simulink model "cc_simulink"  (R2023a)
settings: Solver=VariableStepAuto  StartTime=0.0  StopTime=5100  RelTol=1e-3
undefined symbols (not defined in the file): g_i, g_p
libraries: simulink x6, hdlsllib x1
settings Model: Creator=usradmin  LastModifiedBy=harry

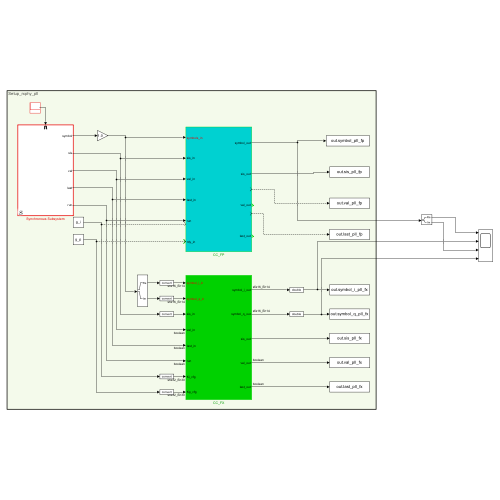
[thumbnail: Simulink's stored preview of the top-level diagram]
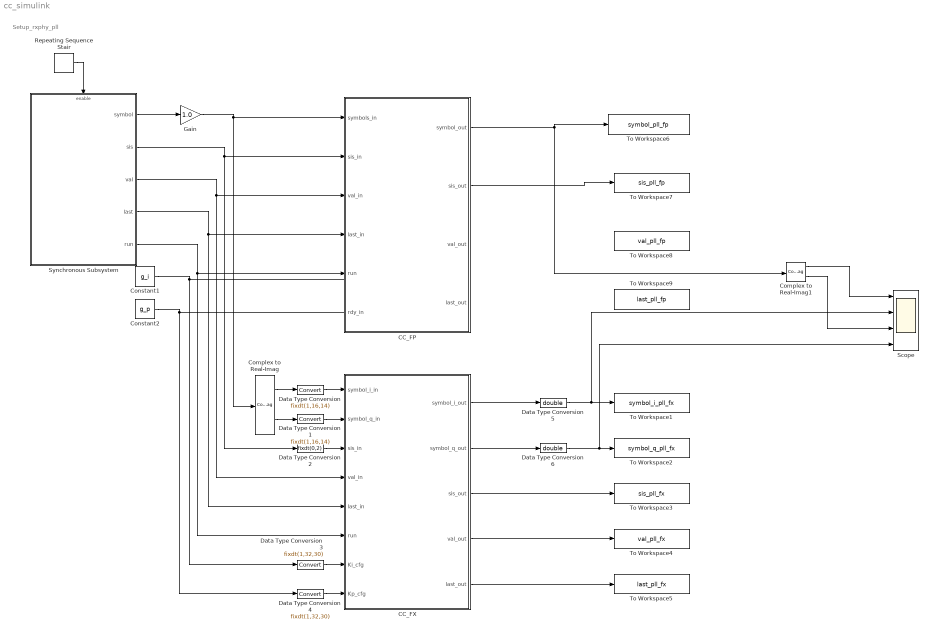
== system cc_simulink ==
  note: Setup_rxphy_pll
  CC_FP : Subsystem
  CC_FX : Subsystem
  Complex to Real-Imag : ComplexToRealImag
  Complex to Real-Imag1 : ComplexToRealImag
  Constant1 : Constant  Value=g_i  SampleTime=-1
  Constant2 : Constant  Value=g_p  SampleTime=-1
  Data Type Conversion : DataTypeConversion  OutDataTypeStr=fixdt(1,16,14)  SaturateOnIntegerOverflow=off  RndMeth=Floor
  Data Type Conversion1 : DataTypeConversion  OutDataTypeStr=fixdt(1,16,14)  SaturateOnIntegerOverflow=off  RndMeth=Floor
  Data Type Conversion2 : DataTypeConversion  OutMin=[0]  OutMax=[3]  OutDataTypeStr=fixdt(0,2)  SaturateOnIntegerOverflow=off  RndMeth=Floor
  Data Type Conversion3 : DataTypeConversion  OutDataTypeStr=fixdt(1,32,30)  SaturateOnIntegerOverflow=off  RndMeth=Floor
  Data Type Conversion4 : DataTypeConversion  OutDataTypeStr=fixdt(1,32,30)  SaturateOnIntegerOverflow=off  RndMeth=Floor
  Data Type Conversion5 : DataTypeConversion  OutDataTypeStr=double  SaturateOnIntegerOverflow=off  RndMeth=Floor
  Data Type Conversion6 : DataTypeConversion  OutDataTypeStr=double  SaturateOnIntegerOverflow=off  RndMeth=Floor
  Gain : Gain  Gain=1.0
  Repeating Sequence Stair : simulink/Sources/Repeating Sequence Stair  OutValues=1  tsamp=1  OutMin=[]  OutMax=[]  OutDataTypeStr=double  OutputDataTypeScalingMode=double  OutDataType=fixdt(0,8)  ConRadixGroup=Best Precision: Vector-wise  OutScaling=2^-12
  Scope : Scope  NumInputPorts=4
  Synchronous Subsystem : Subsystem
  To Workspace1 : ToWorkspace  VariableName=symbol_i_pll_fx  SampleTime=-1
      settings: Save2DSignal=2-D array (concatenate along first dimension)
  To Workspace2 : ToWorkspace  VariableName=symbol_q_pll_fx  SampleTime=-1
      settings: Save2DSignal=2-D array (concatenate along first dimension)
  To Workspace3 : ToWorkspace  VariableName=sis_pll_fx  SampleTime=-1
      settings: Save2DSignal=2-D array (concatenate along first dimension)
  To Workspace4 : ToWorkspace  VariableName=val_pll_fx  SampleTime=-1
      settings: Save2DSignal=2-D array (concatenate along first dimension)
  To Workspace5 : ToWorkspace  VariableName=last_pll_fx  SampleTime=-1
      settings: Save2DSignal=2-D array (concatenate along first dimension)
  To Workspace6 : ToWorkspace  VariableName=symbol_pll_fp  SampleTime=-1
      settings: Save2DSignal=2-D array (concatenate along first dimension)
  To Workspace7 : ToWorkspace  VariableName=sis_pll_fp  SampleTime=-1
      settings: Save2DSignal=2-D array (concatenate along first dimension)
  To Workspace8 : ToWorkspace  VariableName=val_pll_fp  SampleTime=-1
      settings: Save2DSignal=2-D array (concatenate along first dimension)
  To Workspace9 : ToWorkspace  VariableName=last_pll_fp  SampleTime=-1
      settings: Save2DSignal=2-D array (concatenate along first dimension)
  wires:
  Repeating Sequence Stair/1 -> Synchronous Subsystem/Enable
  Synchronous Subsystem/1(symbol) -> Gain/1
  Synchronous Subsystem/4(last) -> CC_FX/5(last_in), CC_FP/4(last_in)
  ? -> To Workspace8/1
  ? -> To Workspace9/1
  Constant1/1 -> Data Type Conversion3/1
  Constant2/1 -> Data Type Conversion4/1
  Synchronous Subsystem/2(sis) -> Data Type Conversion2/1, CC_FP/2(sis_in)
  Synchronous Subsystem/5(run) -> CC_FX/6(run), CC_FP/5(run)
  Synchronous Subsystem/3(val) -> CC_FX/4(val_in), CC_FP/3(val_in)
  CC_FP/2(sis_out) -> To Workspace7/1
  CC_FP/1(symbol_out) -> Complex to Real-Imag1/1, To Workspace6/1
  Data Type Conversion3/1 -> CC_FX/7(Ki_cfg)
  Data Type Conversion4/1 -> CC_FX/8(Kp_cfg)
  Data Type Conversion/1 -> CC_FX/1(symbol_i_in)
  Data Type Conversion1/1 -> CC_FX/2(symbol_q_in)
  Data Type Conversion2/1 -> CC_FX/3(sis_in)
  Complex to Real-Imag/1 -> Data Type Conversion/1
  Complex to Real-Imag/2 -> Data Type Conversion1/1
  CC_FX/1(symbol_i_out) -> Data Type Conversion5/1
  Data Type Conversion5/1 -> Scope/2, To Workspace1/1
  CC_FX/2(symbol_q_out) -> Data Type Conversion6/1
  Data Type Conversion6/1 -> Scope/4, To Workspace2/1
  CC_FX/3(sis_out) -> To Workspace3/1
  CC_FX/4(val_out) -> To Workspace4/1
  CC_FX/5(last_out) -> To Workspace5/1
  Gain/1 -> Complex to Real-Imag/1, CC_FP/1(symbols_in)
  Complex to Real-Imag1/1 -> Scope/1
  Complex to Real-Imag1/2 -> Scope/3

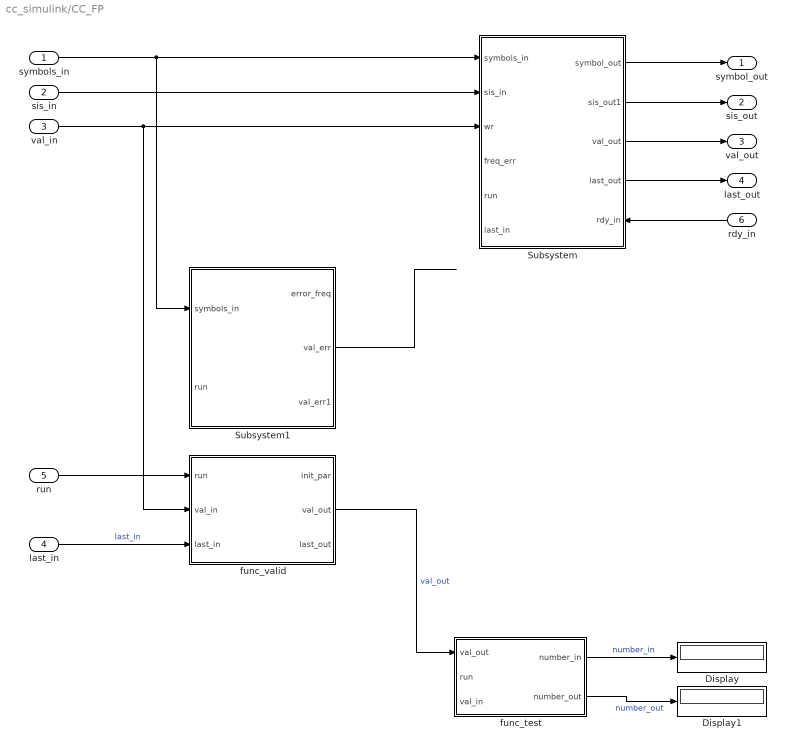
== system cc_simulink/CC_FP ==
  symbols_in : Inport
  sis_in : Inport  Port=2
  val_in : Inport  Port=3
  last_in : Inport  Port=4
  run : Inport  Port=5
  rdy_in : Inport  Port=6
  Display : Display
  Display1 : Display
  Subsystem : Subsystem
      settings: PortSchema="{\"entries\":[{\"content\":{\"sides\":[{\"content\":{\"connectorIds\":[\"In1\",\"In2\",\"In3\",\"In4\",\"In5\",\"In6\"]},\"type\":\"ConnectorPlacement.EquallySpacedRectSide\",\"uuid\":\"c7939d33-c946-4bf1-9bdf-2b3408225bc2\"},{\"content\":{\"connectorIds\":[\"Out1\",\"Out2\",\"Out3\",\"Out4\",\"In7\"],\"side\":\"RIGHT\"},\"type\":\"ConnectorPlacement.EquallySpacedRectSide\",\"uuid\":\"307b9761-00b9-4204-91fa-5162dfa483c4\"},{\"content\":{\"side\":\"TOP\"},\"type\":\"ConnectorPlacement.EquallySpacedRectSide\",\"uuid\":\"84444ae4-1671-4931-bee6-6f05b65457b7\"}]},\"type\":\"ConnectorPlacement.EquallySpacedConnector\",\"uuid\":\"d9ea343b-4c68-49a2-bcf3-6268f7ae1a01\"}],\"packageUris\":[\"http://schema.mathworks.com/mf0/Connector/R2020b\"],\"version\":\"1.0\"}"
  Subsystem1 : Subsystem
  func_test : MATLAB Function  TreatAsAtomicUnit=on
  func_valid : MATLAB Function  TreatAsAtomicUnit=on
  symbol_out : Outport
  sis_out : Outport  Port=2
  val_out : Outport  Port=3
  last_out : Outport  Port=4
  wires:
  val_in/1 -> func_valid/2(val_in), Subsystem/3(wr)
  last_in/1 -> func_valid/3(last_in)  "last_in"
  func_valid/2(val_out) -> func_test/1(val_out)  "val_out"
  run/1 -> func_valid/1(run)
  func_test/1(number_in) -> Display/1  "number_in"
  func_test/2(number_out) -> Display1/1  "number_out"
  symbols_in/1 -> Subsystem1/1(symbols_in), Subsystem/1(symbols_in)
  sis_in/1 -> Subsystem/2(sis_in)
  Subsystem/2(sis_out1) -> sis_out/1
  Subsystem1/2(val_err) -> ?
  Subsystem/1(symbol_out) -> symbol_out/1
  Subsystem/3(val_out) -> val_out/1
  Subsystem/4(last_out) -> last_out/1
  rdy_in/1 -> Subsystem/7(rdy_in)

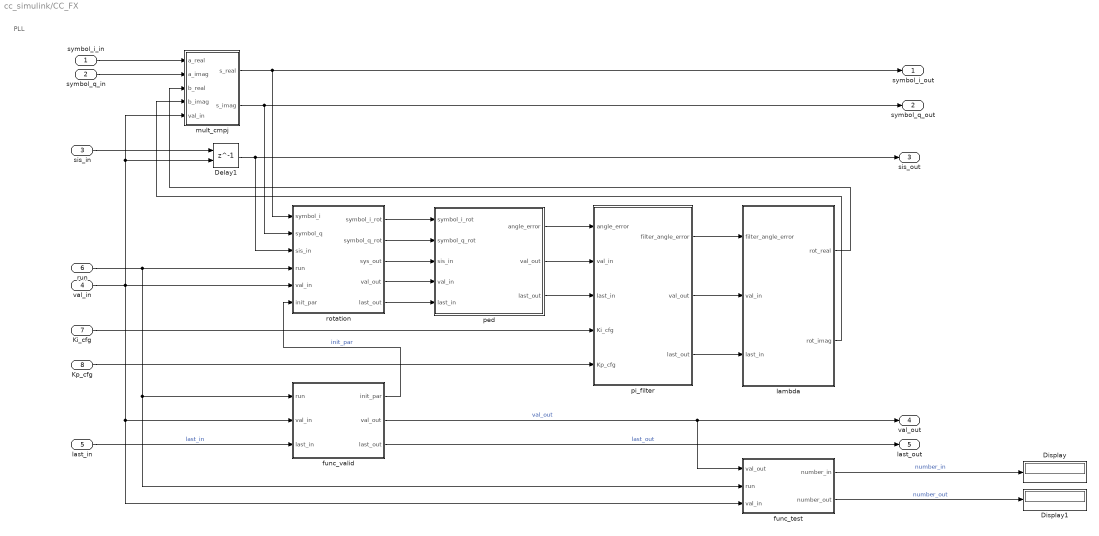
== system cc_simulink/CC_FX ==
  note: PLL
  symbol_i_in : Inport  OutDataTypeStr=fixdt(1,16,14)
  symbol_q_in : Inport  Port=2  OutDataTypeStr=fixdt(1,16,14)
  sis_in : Inport  Port=3  OutMin=[0]  OutMax=[3]  OutDataTypeStr=fixdt(0,2)
  val_in : Inport  Port=4  OutDataTypeStr=boolean
  last_in : Inport  Port=5  OutDataTypeStr=boolean
  run : Inport  Port=6  OutDataTypeStr=boolean
  Ki_cfg : Inport  Port=7  OutDataTypeStr=fixdt(1,32,30)
  Kp_cfg : Inport  Port=8  OutDataTypeStr=fixdt(1,32,30)
  Delay1 : Delay  DelayLength=1  InitialCondition=0  ShowEnablePort=on
      settings: InputPortMap=u0,e6
  Display : Display
  Display1 : Display
  func_test : MATLAB Function  TreatAsAtomicUnit=on
  func_valid : MATLAB Function  TreatAsAtomicUnit=on
  lambda : Subsystem
  mult_cmpj : Subsystem
  ped : Subsystem
  pi_filter : Subsystem
  rotation : Subsystem
  symbol_i_out : Outport  OutDataTypeStr=fixdt(1,16,14)
  symbol_q_out : Outport  Port=2  OutDataTypeStr=fixdt(1,16,14)
  sis_out : Outport  Port=3  OutMin=[0]  OutMax=[3]  OutDataTypeStr=fixdt(0,2)
  val_out : Outport  Port=4  OutDataTypeStr=boolean
  last_out : Outport  Port=5  OutDataTypeStr=boolean
  wires:
  func_test/2(number_out) -> Display1/1  "number_out"
  func_test/1(number_in) -> Display/1  "number_in"
  symbol_i_in/1 -> mult_cmpj/1(a_real)
  func_valid/1(init_par) -> rotation/6(init_par)  "init_par"
  Delay1/1 -> rotation/3(sis_in), sis_out/1
  run/1 -> rotation/4(run), func_valid/1(run), func_test/2(run)
  Kp_cfg/1 -> pi_filter/5(Kp_cfg)
  Ki_cfg/1 -> pi_filter/4(Ki_cfg)
  func_valid/3(last_out) -> last_out/1  "last_out"
  func_valid/2(val_out) -> func_test/1(val_out), val_out/1  "val_out"
  mult_cmpj/1(s_real) -> rotation/1(symbol_i), symbol_i_out/1
  pi_filter/3(last_out) -> lambda/3(last_in)
  pi_filter/2(val_out) -> lambda/2(val_in)
  ped/3(last_out) -> pi_filter/3(last_in)
  ped/2(val_out) -> pi_filter/2(val_in)
  rotation/5(last_out) -> ped/5(last_in)
  rotation/4(val_out) -> ped/4(val_in)
  last_in/1 -> func_valid/3(last_in)  "last_in"
  val_in/1 -> mult_cmpj/5(val_in), Delay1/2, rotation/5(val_in), func_valid/2(val_in), func_test/3(val_in)
  rotation/3(sys_out) -> ped/3(sis_in)
  sis_in/1 -> Delay1/1
  pi_filter/1(filter_angle_error) -> lambda/1(filter_angle_error)
  ped/1(angle_error) -> pi_filter/1(angle_error)
  symbol_q_in/1 -> mult_cmpj/2(a_imag)
  mult_cmpj/2(s_imag) -> symbol_q_out/1, rotation/2(symbol_q)
  rotation/1(symbol_i_rot) -> ped/1(symbol_i_rot)
  rotation/2(symbol_q_rot) -> ped/2(symbol_q_rot)
  lambda/1(rot_real) -> mult_cmpj/3(b_real)
  lambda/2(rot_imag) -> mult_cmpj/4(b_imag)

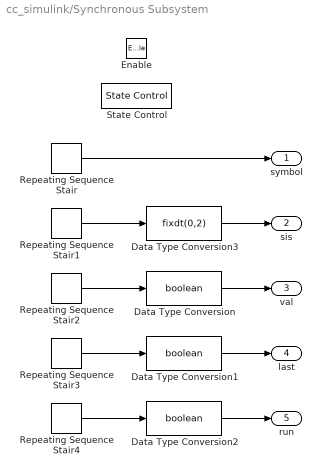
== system cc_simulink/Synchronous Subsystem ==
  Enable : EnablePort  ShowOutputPort=on
  Data Type Conversion : DataTypeConversion  OutDataTypeStr=boolean  SaturateOnIntegerOverflow=off  RndMeth=Floor
  Data Type Conversion1 : DataTypeConversion  OutDataTypeStr=boolean  SaturateOnIntegerOverflow=off  RndMeth=Floor
  Data Type Conversion2 : DataTypeConversion  OutDataTypeStr=boolean  SaturateOnIntegerOverflow=off  RndMeth=Floor
  Data Type Conversion3 : DataTypeConversion  OutMin=[0]  OutMax=[3]  OutDataTypeStr=fixdt(0,2)  SaturateOnIntegerOverflow=off  RndMeth=Floor
  Repeating Sequence Stair : simulink/Sources/Repeating Sequence Stair  OutValues=symbols_cc  tsamp=1  OutMin=[]  OutMax=[]  OutDataTypeStr=double  OutputDataTypeScalingMode=double  OutDataType=fixdt(0,8)  ConRadixGroup=Best Precision: Vector-wise  OutScaling=2^-12
  Repeating Sequence Stair1 : simulink/Sources/Repeating Sequence Stair  OutValues=sis_cc  tsamp=1  OutMin=[]  OutMax=[]  OutDataTypeStr=double  OutputDataTypeScalingMode=double  OutDataType=fixdt(0,8)  ConRadixGroup=Best Precision: Vector-wise  OutScaling=2^-12
  Repeating Sequence Stair2 : simulink/Sources/Repeating Sequence Stair  OutValues=val_cc  tsamp=1  OutMin=[]  OutMax=[]  OutDataTypeStr=double  OutputDataTypeScalingMode=double  OutDataType=fixdt(0,8)  ConRadixGroup=Best Precision: Vector-wise  OutScaling=2^-12
  Repeating Sequence Stair3 : simulink/Sources/Repeating Sequence Stair  OutValues=last_cc  tsamp=1  OutMin=[]  OutMax=[]  OutDataTypeStr=double  OutputDataTypeScalingMode=double  OutDataType=fixdt(0,8)  ConRadixGroup=Best Precision: Vector-wise  OutScaling=2^-12
  Repeating Sequence Stair4 : simulink/Sources/Repeating Sequence Stair  OutValues=run_cc  tsamp=1  OutMin=[]  OutMax=[]  OutDataTypeStr=double  OutputDataTypeScalingMode=double  OutDataType=fixdt(0,8)  ConRadixGroup=Best Precision: Vector-wise  OutScaling=2^-12
  State Control : StateControl  StateControl=Synchronous
  symbol : Outport  VectorParamsAs1DForOutWhenUnconnected=off
  sis : Outport  Port=2  VectorParamsAs1DForOutWhenUnconnected=off
  val : Outport  Port=3  VectorParamsAs1DForOutWhenUnconnected=off
  last : Outport  Port=4  VectorParamsAs1DForOutWhenUnconnected=off
  run : Outport  Port=5  VectorParamsAs1DForOutWhenUnconnected=off
  wires:
  Repeating Sequence Stair/1 -> symbol/1
  Repeating Sequence Stair1/1 -> Data Type Conversion3/1
  Repeating Sequence Stair3/1 -> Data Type Conversion1/1
  Repeating Sequence Stair2/1 -> Data Type Conversion/1
  Repeating Sequence Stair4/1 -> Data Type Conversion2/1
  Data Type Conversion/1 -> val/1
  Data Type Conversion1/1 -> last/1
  Data Type Conversion2/1 -> run/1
  Data Type Conversion3/1 -> sis/1

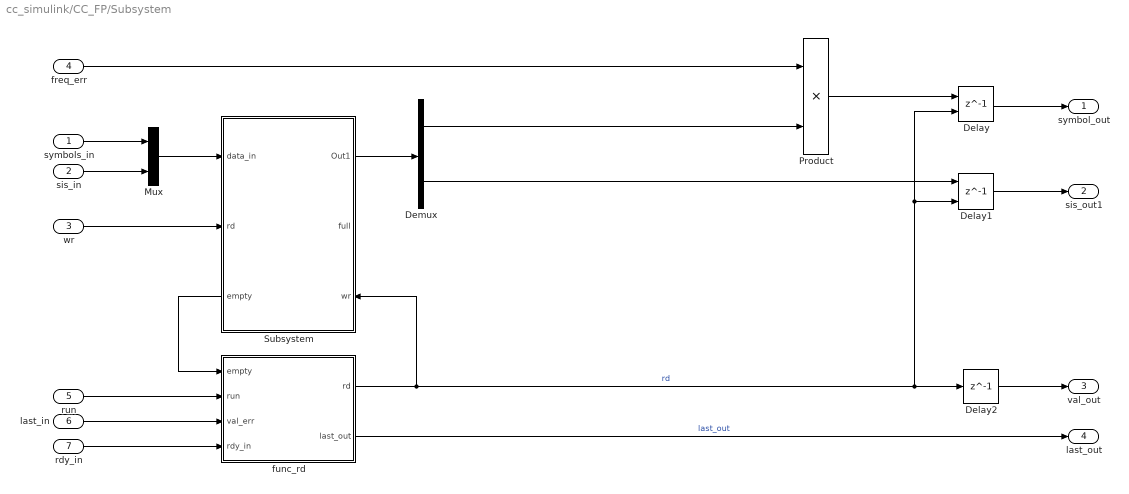
== system cc_simulink/CC_FP/Subsystem ==
  symbols_in : Inport
  sis_in : Inport  Port=2
  wr : Inport  Port=3
  freq_err : Inport  Port=4
  run : Inport  Port=5
  last_in : Inport  Port=6
  rdy_in : Inport  Port=7
  Delay : Delay  DelayLength=1  InitialCondition=0  ShowEnablePort=on
      settings: InputPortMap=u0,e6
  Delay1 : Delay  DelayLength=1  InitialCondition=0  ShowEnablePort=on
      settings: InputPortMap=u0,e6
  Delay2 : Delay  DelayLength=1  InitialCondition=0
  Demux : Demux  Outputs=2
  Mux : Mux  Inputs=2
  Product : Product
  Subsystem : Subsystem
      settings: PortSchema="{\"entries\":[{\"content\":{\"sides\":[{\"content\":{\"connectorIds\":[\"In1\",\"In2\",\"Out3\"]},\"type\":\"ConnectorPlacement.EquallySpacedRectSide\",\"uuid\":\"bfd53dd1-7a31-4f51-b3c2-6d63477d1785\"},{\"content\":{\"connectorIds\":[\"Out1\",\"Out2\",\"In3\"],\"side\":\"RIGHT\"},\"type\":\"ConnectorPlacement.EquallySpacedRectSide\",\"uuid\":\"4f2d7eeb-26ef-45c7-bd9a-3a631e6797b8\"},{\"content\":{\"side\":\"TOP\"},\"type\":\"ConnectorPlacement.EquallySpacedRectSide\",\"uuid\":\"17e64bb6-dd6a-4970-b765-577857b607e2\"}]},\"type\":\"ConnectorPlacement.EquallySpacedConnector\",\"uuid\":\"4ca766b8-8fb8-4689-a29d-3d913e337836\"}],\"packageUris\":[\"http://schema.mathworks.com/mf0/Connector/R2020b\"],\"version\":\"1.0\"}"
  func_rd : MATLAB Function  TreatAsAtomicUnit=on
  symbol_out : Outport
  sis_out1 : Outport  Port=2
  val_out : Outport  Port=3
  last_out : Outport  Port=4
  wires:
  symbols_in/1 -> Mux/1
  sis_in/1 -> Mux/2
  Delay2/1 -> val_out/1
  Delay1/1 -> sis_out1/1
  Product/1 -> Delay/1
  Demux/2 -> Delay1/1
  Delay/1 -> symbol_out/1
  func_rd/1(rd) -> Subsystem/3(wr), Delay/2, Delay1/2, Delay2/1  "rd"
  Demux/1 -> Product/2
  freq_err/1 -> Product/1
  run/1 -> func_rd/2(run)
  func_rd/2(last_out) -> last_out/1  "last_out"
  Mux/1 -> Subsystem/1(data_in)
  wr/1 -> Subsystem/2(rd)
  Subsystem/1(Out1) -> Demux/1
  Subsystem/3(empty) -> func_rd/1(empty)
  last_in/1 -> func_rd/3(val_err)
  rdy_in/1 -> func_rd/4(rdy_in)

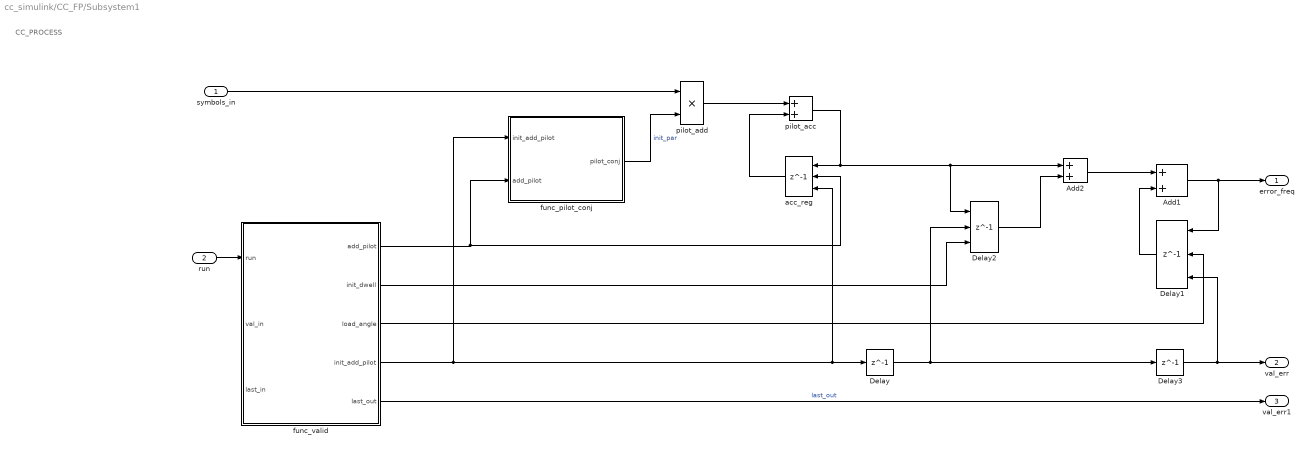
== system cc_simulink/CC_FP/Subsystem1 ==
  note: CC_PROCESS
  symbols_in : Inport
  run : Inport  Port=2
  Add1 : Sum
  Add2 : Sum
  Delay : Delay  DelayLength=1  InitialCondition=0
  Delay1 : Delay  DelayLength=1  InitialCondition=0  ExternalReset=Level  ShowEnablePort=on
      settings: InputPortMap=u0,e6,r5
  Delay2 : Delay  DelayLength=1  InitialCondition=0  ExternalReset=Level  ShowEnablePort=on
      settings: InputPortMap=u0,e6,r5
  Delay3 : Delay  DelayLength=1  InitialCondition=0
  acc_reg : Delay  DelayLength=1  InitialCondition=0  ExternalReset=Level  ShowEnablePort=on
      settings: InputPortMap=u0,e6,r5
  func_pilot_conj : MATLAB Function  TreatAsAtomicUnit=on
  func_valid : MATLAB Function  TreatAsAtomicUnit=on
  pilot_acc : Sum
  pilot_add : Product
  error_freq : Outport
  val_err : Outport  Port=2
  val_err1 : Outport  Port=3
  wires:
  pilot_acc/1 -> Add2/1, Delay2/1, acc_reg/1
  Delay2/1 -> Add2/2
  Delay1/1 -> Add1/2
  Add1/1 -> Delay1/1, error_freq/1
  Add2/1 -> Add1/1
  acc_reg/1 -> pilot_acc/2
  func_valid/1(add_pilot) -> func_pilot_conj/2(add_pilot), acc_reg/2
  func_valid/3(load_angle) -> Delay1/2
  func_valid/4(init_add_pilot) -> acc_reg/3, Delay/1, func_pilot_conj/1(init_add_pilot)
  symbols_in/1 -> pilot_add/1
  pilot_add/1 -> pilot_acc/1
  func_pilot_conj/1(pilot_conj) -> pilot_add/2  "init_par"
  Delay/1 -> Delay3/1, Delay2/2
  func_valid/2(init_dwell) -> Delay2/3
  Delay3/1 -> val_err/1, Delay1/3
  run/1 -> func_valid/1(run)
  func_valid/5(last_out) -> val_err1/1  "last_out"

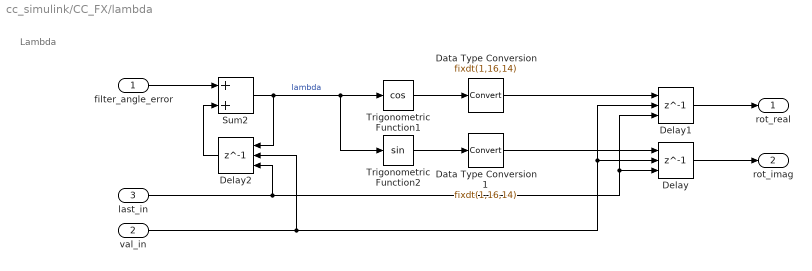
== system cc_simulink/CC_FX/lambda ==
  note: Lambda
  filter_angle_error : Inport
  val_in : Inport  Port=2
  last_in : Inport  Port=3
  Data Type Conversion : DataTypeConversion  OutDataTypeStr=fixdt(1,16,14)  SaturateOnIntegerOverflow=off  RndMeth=Floor
  Data Type Conversion1 : DataTypeConversion  OutDataTypeStr=fixdt(1,16,14)  SaturateOnIntegerOverflow=off  RndMeth=Floor
  Delay : Delay  DelayLength=1  InitialCondition=0  ExternalReset=Level  ShowEnablePort=on
      settings: InputPortMap=u0,e6,r5
  Delay1 : Delay  DelayLength=1  InitialCondition=0  ExternalReset=Level  ShowEnablePort=on
      settings: InputPortMap=u0,e6,r5
  Delay2 : Delay  DelayLength=1  ExternalReset=Level  ShowEnablePort=on
      settings: InputPortMap=u0,e6,r5
  Sum2 : Sum  AccumDataTypeStr=fixdt(1,24,20)
  Trigonometric Function1 : Trigonometry  Operator=cos  ApproximationMethod=Lookup  NumberOfDataPoints=2048  TableDataTypeStr=fixdt(1,12,10)
  Trigonometric Function2 : Trigonometry  ApproximationMethod=Lookup  NumberOfDataPoints=4096  TableDataTypeStr=fixdt(1,12,10)
  rot_real : Outport
  rot_imag : Outport  Port=2
  wires:
  Trigonometric Function1/1 -> Data Type Conversion/1
  Trigonometric Function2/1 -> Data Type Conversion1/1
  Delay/1 -> rot_imag/1
  val_in/1 -> Delay2/2, Delay1/2, Delay/2
  last_in/1 -> Delay2/3, Delay1/3, Delay/3
  filter_angle_error/1 -> Sum2/1
  Delay2/1 -> Sum2/2
  Sum2/1 -> Delay2/1, Trigonometric Function2/1, Trigonometric Function1/1  "lambda"
  Data Type Conversion/1 -> Delay1/1
  Data Type Conversion1/1 -> Delay/1
  Delay1/1 -> rot_real/1

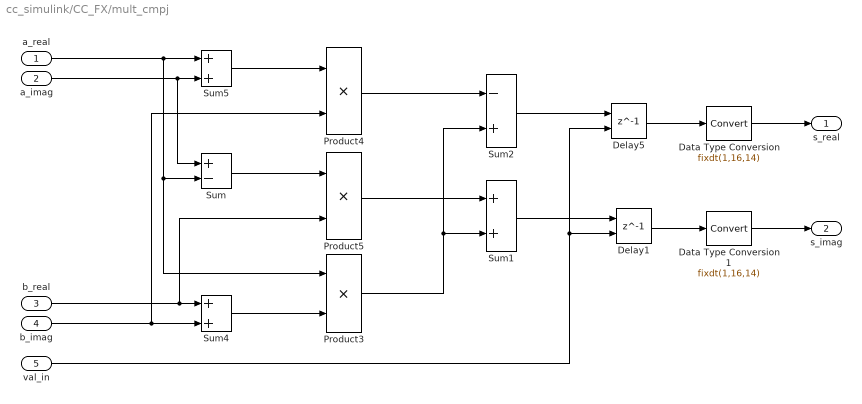
== system cc_simulink/CC_FX/mult_cmpj ==
  a_real : Inport
  a_imag : Inport  Port=2
  b_real : Inport  Port=3
  b_imag : Inport  Port=4
  val_in : Inport  Port=5
  Data Type Conversion : DataTypeConversion  OutDataTypeStr=fixdt(1,16,14)  SaturateOnIntegerOverflow=off  RndMeth=Floor
  Data Type Conversion1 : DataTypeConversion  OutDataTypeStr=fixdt(1,16,14)  SaturateOnIntegerOverflow=off  RndMeth=Floor
  Delay1 : Delay  DelayLength=1  InitialCondition=0  ShowEnablePort=on
      settings: InputPortMap=u0,e6
  Delay5 : Delay  DelayLength=1  InitialCondition=0  ShowEnablePort=on
      settings: InputPortMap=u0,e6
  Product3 : Product
  Product4 : Product
  Product5 : Product
  Sum : Sum  Inputs=+-
  Sum1 : Sum
  Sum2 : Sum  Inputs=-+
  Sum4 : Sum
  Sum5 : Sum
  s_real : Outport
  s_imag : Outport  Port=2
  wires:
  Product3/1 -> Sum1/2, Sum2/2
  Sum1/1 -> Delay1/1
  b_real/1 -> Sum4/1, Product5/2
  Sum2/1 -> Delay5/1
  a_real/1 -> Sum5/1, Product3/1, Sum/2
  b_imag/1 -> Sum4/2, Product4/2
  a_imag/1 -> Sum/1, Sum5/2
  Sum4/1 -> Product3/2
  Sum5/1 -> Product4/1
  Sum/1 -> Product5/1
  Product4/1 -> Sum2/1
  Product5/1 -> Sum1/1
  Delay5/1 -> Data Type Conversion/1
  Delay1/1 -> Data Type Conversion1/1
  val_in/1 -> Delay5/2, Delay1/2
  Data Type Conversion/1 -> s_real/1
  Data Type Conversion1/1 -> s_imag/1

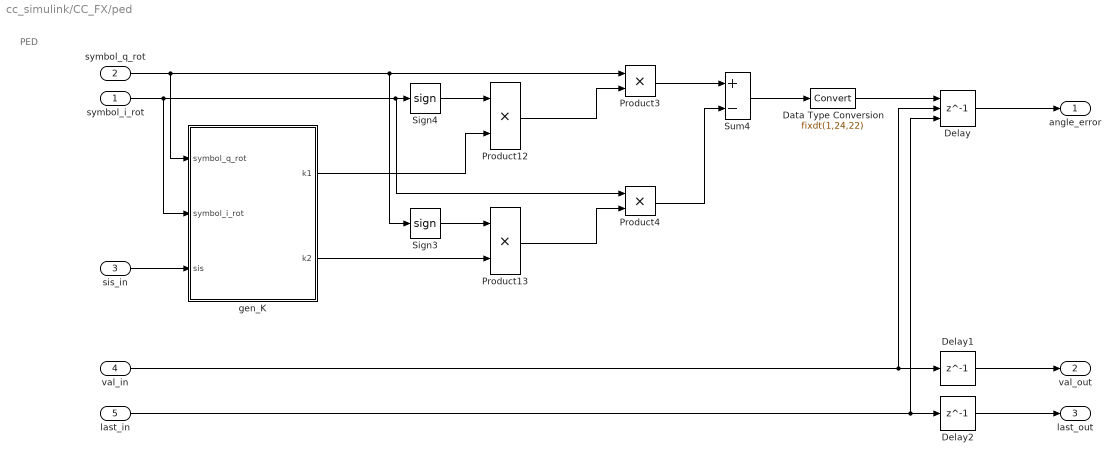
== system cc_simulink/CC_FX/ped ==
  note: PED
  symbol_i_rot : Inport
  symbol_q_rot : Inport  Port=2
  sis_in : Inport  Port=3
  val_in : Inport  Port=4
  last_in : Inport  Port=5
  Data Type Conversion : DataTypeConversion  OutDataTypeStr=fixdt(1,24,22)  SaturateOnIntegerOverflow=off  RndMeth=Floor
  Delay : Delay  DelayLength=1  InitialCondition=0  ExternalReset=Level  ShowEnablePort=on
      settings: InputPortMap=u0,e6,r5
  Delay1 : Delay  DelayLength=1  InitialCondition=0
  Delay2 : Delay  DelayLength=1  InitialCondition=0
  Product{3..4,12..13} (4 alike) : Product
  Sign3 : Signum
  Sign4 : Signum
  Sum4 : Sum  Inputs=+-
  gen_K : MATLAB Function  TreatAsAtomicUnit=on
  angle_error : Outport
  val_out : Outport  Port=2
  last_out : Outport  Port=3
  wires:
  gen_K/2(k2) -> Product13/2
  last_in/1 -> Delay/3, Delay2/1
  val_in/1 -> Delay1/1, Delay/2
  sis_in/1 -> gen_K/3(sis)
  Product13/1 -> Product4/2
  symbol_q_rot/1 -> gen_K/1(symbol_q_rot), Product3/1, Sign3/1
  Sign4/1 -> Product12/1
  Sign3/1 -> Product13/1
  Product4/1 -> Sum4/2
  Sum4/1 -> Data Type Conversion/1
  gen_K/1(k1) -> Product12/2
  Product12/1 -> Product3/2
  Product3/1 -> Sum4/1
  symbol_i_rot/1 -> gen_K/2(symbol_i_rot), Product4/1, Sign4/1
  Delay/1 -> angle_error/1
  Delay1/1 -> val_out/1
  Delay2/1 -> last_out/1
  Data Type Conversion/1 -> Delay/1

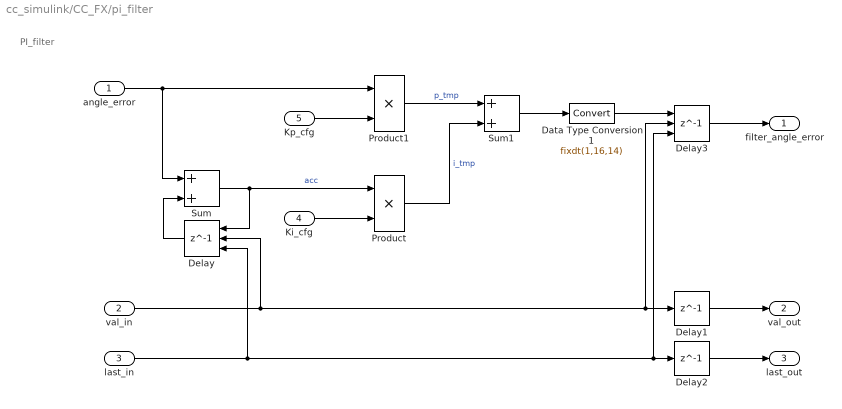
== system cc_simulink/CC_FX/pi_filter ==
  note: PI_filter
  angle_error : Inport
  val_in : Inport  Port=2
  last_in : Inport  Port=3
  Ki_cfg : Inport  Port=4
  Kp_cfg : Inport  Port=5
  Data Type Conversion1 : DataTypeConversion  OutDataTypeStr=fixdt(1,16,14)  SaturateOnIntegerOverflow=off  RndMeth=Floor
  Delay : Delay  DelayLength=1  ExternalReset=Level  ShowEnablePort=on
      settings: InputPortMap=u0,e6,r5
  Delay1 : Delay  DelayLength=1  InitialCondition=0
  Delay2 : Delay  DelayLength=1  InitialCondition=0
  Delay3 : Delay  DelayLength=1  InitialCondition=0  ExternalReset=Level  ShowEnablePort=on
      settings: InputPortMap=u0,e6,r5
  Product : Product  OutDataTypeStr=fixdt(1,48,44)
  Product1 : Product
  Sum : Sum  AccumDataTypeStr=fixdt(1,32,24)
  Sum1 : Sum
  filter_angle_error : Outport
  val_out : Outport  Port=2
  last_out : Outport  Port=3
  wires:
  Sum1/1 -> Data Type Conversion1/1
  Kp_cfg/1 -> Product1/2
  Ki_cfg/1 -> Product/2
  last_in/1 -> Delay3/3, Delay2/1, Delay/3
  val_in/1 -> Delay3/2, Delay1/1, Delay/2
  Product/1 -> Sum1/2  "i_tmp"
  angle_error/1 -> Product1/1, Sum/1
  Product1/1 -> Sum1/1  "p_tmp"
  Delay/1 -> Sum/2
  Sum/1 -> Product/1, Delay/1  "acc"
  Delay1/1 -> val_out/1
  Delay2/1 -> last_out/1
  Delay3/1 -> filter_angle_error/1
  Data Type Conversion1/1 -> Delay3/1

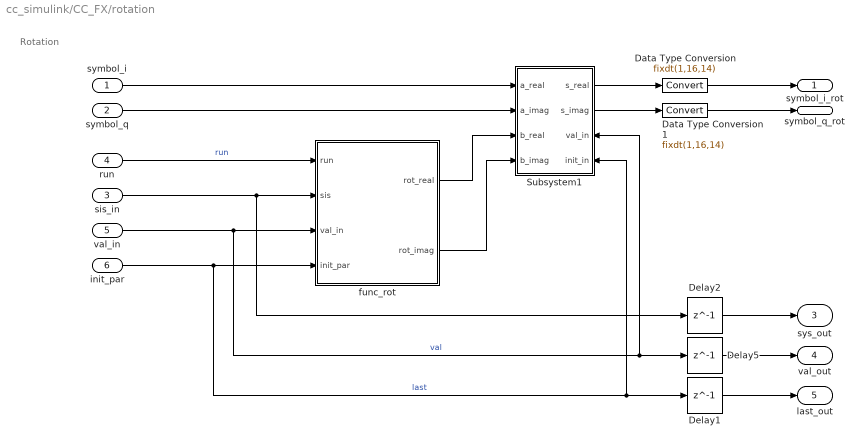
== system cc_simulink/CC_FX/rotation ==
  note: Rotation
  symbol_i : Inport
  symbol_q : Inport  Port=2
  sis_in : Inport  Port=3
  run : Inport  Port=4
  val_in : Inport  Port=5
  init_par : Inport  Port=6
  Data Type Conversion : DataTypeConversion  OutDataTypeStr=fixdt(1,16,14)  SaturateOnIntegerOverflow=off  RndMeth=Floor
  Data Type Conversion1 : DataTypeConversion  OutDataTypeStr=fixdt(1,16,14)  SaturateOnIntegerOverflow=off  RndMeth=Floor
  Delay1 : Delay  DelayLength=1  InitialCondition=0
  Delay2 : Delay  DelayLength=1  InitialCondition=0
  Delay5 : Delay  DelayLength=1  InitialCondition=0
  Subsystem1 : Subsystem
      settings: PortSchema="{\"entries\":[{\"content\":{\"sides\":[{\"content\":{\"connectorIds\":[\"In1\",\"In2\",\"In3\",\"In4\"]},\"type\":\"ConnectorPlacement.EquallySpacedRectSide\",\"uuid\":\"87a88ef2-5145-45be-b41f-bbadaafc86ad\"},{\"content\":{\"connectorIds\":[\"Out1\",\"Out2\",\"In5\",\"In6\"],\"side\":\"RIGHT\"},\"type\":\"ConnectorPlacement.EquallySpacedRectSide\",\"uuid\":\"f2bc7072-b2a3-4904-b872-3606352800dc\"},{\"content\":{\"side\":\"TOP\"},\"type\":\"ConnectorPlacement.EquallySpacedRectSide\",\"uuid\":\"6770ae99-0d9f-4d99-9379-c512154f11d6\"}]},\"type\":\"ConnectorPlacement.EquallySpacedConnector\",\"uuid\":\"93acd5ab-1ba3-475e-82e0-c8dad4706105\"}],\"packageUris\":[\"http://schema.mathworks.com/mf0/Connector/R2020b\"],\"version\":\"1.0\"}"
  func_rot : MATLAB Function  TreatAsAtomicUnit=on
  symbol_i_rot : Outport
  symbol_q_rot : Outport  Port=2
  sys_out : Outport  Port=3
  val_out : Outport  Port=4
  last_out : Outport  Port=5
  wires:
  run/1 -> func_rot/1(run)  "run"
  sis_in/1 -> Delay2/1, func_rot/2(sis)
  init_par/1 -> Subsystem1/6(init_in), Delay1/1, func_rot/4(init_par)  "last"
  val_in/1 -> Subsystem1/5(val_in), Delay5/1, func_rot/3(val_in)  "val"
  func_rot/1(rot_real) -> Subsystem1/3(b_real)
  Subsystem1/1(s_real) -> Data Type Conversion/1
  func_rot/2(rot_imag) -> Subsystem1/4(b_imag)
  Subsystem1/2(s_imag) -> Data Type Conversion1/1
  symbol_q/1 -> Subsystem1/2(a_imag)
  symbol_i/1 -> Subsystem1/1(a_real)
  Delay5/1 -> val_out/1
  Delay1/1 -> last_out/1
  Delay2/1 -> sys_out/1
  Data Type Conversion/1 -> symbol_i_rot/1
  Data Type Conversion1/1 -> symbol_q_rot/1

== system cc_simulink/CC_FP/Subsystem/Subsystem ==
  data_in : Inport
  rd : Inport  Port=2
  wr : Inport  Port=3
  fifo_in : hdlsllib/HDL RAMs/HDL FIFO  fifo_size=1024  mode=Classic  ratio=1  push_msg=Warning  pop_msg=Warning  show_empty=on  show_full=on  show_num=on  LabelModeActiveChoice_Mode=Classic  rst_port=off
  Out1 : Outport
  full : Outport  Port=2
  empty : Outport  Port=3
  wires:
  wr/1 -> fifo_in/3
  fifo_in/3 -> full/1
  rd/1 -> fifo_in/2
  fifo_in/2 -> empty/1
  data_in/1 -> fifo_in/1
  fifo_in/1 -> Out1/1

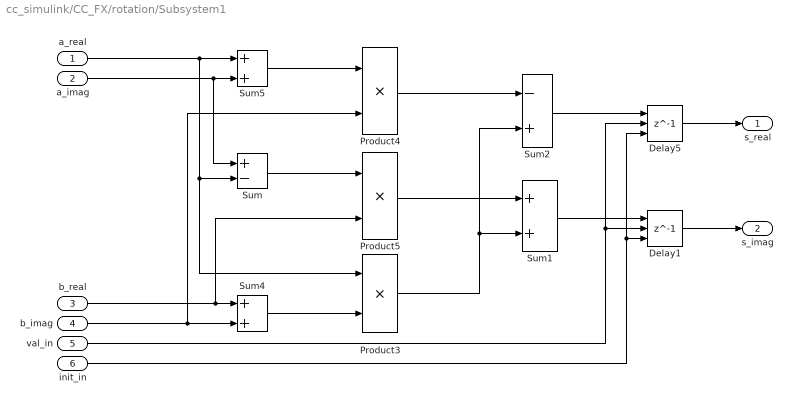
== system cc_simulink/CC_FX/rotation/Subsystem1 ==
  a_real : Inport
  a_imag : Inport  Port=2
  b_real : Inport  Port=3
  b_imag : Inport  Port=4
  val_in : Inport  Port=5
  init_in : Inport  Port=6
  Delay1 : Delay  DelayLength=1  InitialCondition=0  ExternalReset=Level  ShowEnablePort=on
      settings: InputPortMap=u0,e6,r5
  Delay5 : Delay  DelayLength=1  InitialCondition=0  ExternalReset=Level  ShowEnablePort=on
      settings: InputPortMap=u0,e6,r5
  Product3 : Product
  Product4 : Product
  Product5 : Product
  Sum : Sum  Inputs=+-
  Sum1 : Sum
  Sum2 : Sum  Inputs=-+
  Sum4 : Sum
  Sum5 : Sum
  s_real : Outport
  s_imag : Outport  Port=2
  wires:
  Product3/1 -> Sum1/2, Sum2/2
  Sum1/1 -> Delay1/1
  b_real/1 -> Sum4/1, Product5/2
  Sum2/1 -> Delay5/1
  a_real/1 -> Sum5/1, Product3/1, Sum/2
  b_imag/1 -> Sum4/2, Product4/2
  a_imag/1 -> Sum/1, Sum5/2
  Sum4/1 -> Product3/2
  Sum5/1 -> Product4/1
  Sum/1 -> Product5/1
  Product4/1 -> Sum2/1
  Product5/1 -> Sum1/1
  Delay5/1 -> s_real/1
  Delay1/1 -> s_imag/1
  val_in/1 -> Delay5/2, Delay1/2
  init_in/1 -> Delay5/3, Delay1/3

== matlab function cc_simulink/CC_FP/Subsystem1/func_valid ==
  data: add_pilot output; init_dwell output; load_angle output; init_add_pilot output; run input; val_in input; last_in input; last_out output
function [add_pilot, init_dwell, load_angle, init_add_pilot,  last_out] = func_valid(run, val_in, last_in)
% -------------------------------------------------------------------------
% Function valid
% -------------------------------------------------------------------------
    % persistent variable for the state 
    persistent count;
    if isempty(count)
        count = uint16(0);
    end

    % persistent variable for the state 
    persistent count_dwell;
    if isempty(count_dwell)
        count_dwell = uint8(0);
    end

    persistent add_pilot;
    if isempty(add_pilot)
        add_pilot = false;
    end

    % dwell symbol counter
    if (not(run) || (val_in && (last_in || count > uint16(946))))
         count = uint16(0);
    elseif (val_in)
        count = count + uint16(1);
    end

    % dwell number counter 
    if (not(run) || (val_in && (last_in || count > uint16(946))))
        count_dwell = uint8(0);
    elseif (val_in && count == uint16(946))
        count_dwell = count_dwell + uint8(1);
    end

    % generate the add pilot
    if (not(run) || (val_in && (last_in || count > uint16(946))))
       add_pilot = false; 
    elseif (count == uint16(64+32) || ...
            count == uint16(64+32+11) || ...
            count == uint16(64+32+11+157) || ...
            count == uint16(64+32+11+157+11) || ...
            count == uint16(64+32+11+157+11+157) || ...
            count == uint16(64+32+11+157+11+157+11) || ...
            count == uint16(64+32+11+157+11+157+11+157) || ...
            count == uint16(64+32+11+157+11+157+11+157+11) || ...
            count == uint16(64+32+11+157+11+157+11+157+11+157) || ...
            count == uint16(64+32+11+157+11+157+11+157+11+157+11) || ...
            count == uint16(64+32+11+157+11+157+11+157+11+157+11+157) || ...
            count == uint16(64+32+11+157+11+157+11+157+11+157+11+157+11))

        add_pilot = not(add_pilot);
    end
    

    % calculate last
    if (count_dwell == uint8(4) && count == uint16(935))
        last_out = true;
    else
        last_out = false;
    end

    % calculate last
    if (count == uint16(946) && val_in)
        init_par_int = true;
    else
        init_par_int = false;
    end

    val_out = mask_int && val_in;
    init_par = init_par_int && val_in;

end 
% -------------------------------------------------------------------------

== matlab function cc_simulink/CC_FP/func_valid ==
  data: run input; val_in input; init_par output; last_in input; val_out output; last_out output
function [init_par, val_out, last_out] = func_valid(run, val_in, last_in)
% -------------------------------------------------------------------------
% Function valid
% -------------------------------------------------------------------------
    % persistent variable for the state 
    persistent count;
    if isempty(count)
        count = uint16(0);
    end

    % persistent variable for the state 
    persistent count_dwell;
    if isempty(count_dwell)
        count_dwell = uint8(0);
    end

    persistent add_pilot;
    if isempty(add_pilot)
        add_pilot = false;
    end

    % dwell symbol counter
    if (not(run) || (val_in && (last_in || count > uint16(946))))
         count = uint16(0);
    elseif (val_in)
        count = count + uint16(1);
    end

    % dwell number counter 
    if (not(run) || (val_in && (last_in || count > uint16(946))))
        count_dwell = uint8(0);
    elseif (val_in && count == uint16(946))
        count_dwell = count_dwell + uint8(1);
    end

    % generate the add pilot
    if (not(run) || (val_in && (last_in || count > uint16(946))))
       add_pilot = false; 
    elseif (count == uint16(64+32) || ...
            count == uint16(64+32+11) || ...
            count == uint16(64+32+11+157) || ...
            count == uint16(64+32+11+157+11) || ...
            count == uint16(64+32+11+157+11+157) || ...
            count == uint16(64+32+11+157+11+157+11) || ...
            count == uint16(64+32+11+157+11+157+11+157) || ...
            count == uint16(64+32+11+157+11+157+11+157+11) || ...
            count == uint16(64+32+11+157+11+157+11+157+11+157) || ...
            count == uint16(64+32+11+157+11+157+11+157+11+157+11) || ...
            count == uint16(64+32+11+157+11+157+11+157+11+157+11+157) || ...
            count == uint16(64+32+11+157+11+157+11+157+11+157+11+157+11))

        add_pilot = not(add_pilot);
    end
    

    % calculate last
    if (count_dwell == uint8(4) && count == uint16(935))
        last_out = true;
    else
        last_out = false;
    end

    % calculate last
    if (count == uint16(946) && val_in)
        init_par_int = true;
    else
        init_par_int = false;
    end

    val_out = mask_int && val_in;
    init_par = init_par_int && val_in;

end 
% -------------------------------------------------------------------------

== matlab function cc_simulink/CC_FP/Subsystem1/func_pilot_conj ==
  data: init_add_pilot input; pilot_conj output; add_pilot input
function pilot_conj = func_pilot_conj(init_add_pilot, add_pilot)
% -------------------------------------------------------------------------
% Function valid
% -------------------------------------------------------------------------
    % persistent variable for the state 
    persistent count;
    if isempty(count)
        count = uint8(0);
    end

    % pilot counter
    if (init_add_pilot)
         count = uint8(0);
    elseif (add_pilot)
        count = count + uint8(1);
    end

    % select conjuate pilot
    switch count
        case {0}
            pilot_conj = 1+1i;
        case {1}
            pilot_conj = 1+1i;
        case {2}
            pilot_conj = 1+1i;
        case {3}        
            pilot_conj = 1+1i;
        case {4}        
            pilot_conj = 1+1i;
        case {5}        
            pilot_conj = 1+1i;
        case {6}        
            pilot_conj = 1+1i;
        case {7}        
            pilot_conj = 1+1i;
        case {8}        
            pilot_conj = 1+1i;
        case {9}        
            pilot_conj = 1+1i;
        otherwise
            pilot_conj = 1+1i;
    end

end 
% -------------------------------------------------------------------------

== matlab function cc_simulink/CC_FX/func_test ==
  data: val_out input; run input; val_in input; number_in output; number_out output
function [number_in, number_out] = func_test(val_out, run, val_in)
% -------------------------------------------------------------------------
% Function valid
% -------------------------------------------------------------------------
    % persistent variable for the state 
    persistent count_out;
    if isempty(count_out)
        count_out = uint16(0);
    end

    % counting up
    if (not(run))
        count_out = uint16(0);
    elseif (val_out)
        count_out = count_out + uint16(1);
    end

    number_out = count_out;

    % persistent variable for the state 
    persistent count_in;
    if isempty(count_in)
        count_in = uint16(0);
    end

    % counting up
    if (not(run))
        count_in = uint16(0);
    elseif (val_in)
        count_in = count_in + uint16(1);
    end

    number_in = count_in;
end 
% -------------------------------------------------------------------------

== matlab function cc_simulink/CC_FP/func_test ==
  data: val_out input; run input; val_in input; number_in output; number_out output
function [number_in, number_out] = func_test(val_out, run, val_in)
% -------------------------------------------------------------------------
% Function valid
% -------------------------------------------------------------------------
    % persistent variable for the state 
    persistent count_out;
    if isempty(count_out)
        count_out = uint16(0);
    end

    % counting up
    if (not(run))
        count_out = uint16(0);
    elseif (val_out)
        count_out = count_out + uint16(1);
    end

    number_out = count_out;

    % persistent variable for the state 
    persistent count_in;
    if isempty(count_in)
        count_in = uint16(0);
    end

    % counting up
    if (not(run))
        count_in = uint16(0);
    elseif (val_in)
        count_in = count_in + uint16(1);
    end

    number_in = count_in;
end 
% -------------------------------------------------------------------------

== matlab function cc_simulink/CC_FX/func_valid ==
  data: run input; val_in input; init_par output; last_in input; val_out output; last_out output
function [init_par, val_out, last_out] = func_valid(run, val_in, last_in)
% -------------------------------------------------------------------------
% Function valid
% -------------------------------------------------------------------------
    % persistent variable for the state 
    persistent count;
    if isempty(count)
        count = uint16(0);
    end

    % persistent variable for the state 
    persistent count_dwell;
    if isempty(count_dwell)
        count_dwell = uint8(0);
    end

    persistent mask_int;
    if isempty(mask_int)
        mask_int = false;
    end

    % counting up
    if (not(run))
        count = uint16(0);
    elseif (val_in)
        count = count + uint16(1);
        % limit 
        if (last_in || count > uint16(946))
            count = uint16(0);
        end
    end

    % counting dwell
    if (not(run))
        count_dwell = uint8(0);
    elseif (val_in && count == uint16(946))
        count_dwell = count_dwell + uint8(1);
        % limit to four bits
        if (last_in)
            count_dwell = uint8(0);
        end
    end

    % Calculate the mask
    if (count == uint16(107) || ...
        count == uint16(107+157) || ...
        count == uint16(107+157+11) || ...
        count == uint16(107+157+11+157) || ...
        count == uint16(107+157+11+157+11) || ...
        count == uint16(107+157+11+157+11+157) || ...
        count == uint16(107+157+11+157+11+157+11) || ...
        count == uint16(107+157+11+157+11+157+11+157) || ...
        count == uint16(107+157+11+157+11+157+11+157+11) || ...
        count == uint16(107+157+11+157+11+157+11+157+11+157))
        mask_int = not(mask_int);
    end

    % calculate last
    if (count_dwell == uint8(4) && count == uint16(935))
        last_out = true;
    else
        last_out = false;
    end

    % calculate last
    if (count == uint16(946) && val_in)
        init_par_int = true;
    else
        init_par_int = false;
    end

    val_out = mask_int && val_in;
    init_par = init_par_int && val_in;

end 
% -------------------------------------------------------------------------

== matlab function cc_simulink/CC_FX/ped/gen_K ==
  data: symbol_q_rot input; symbol_i_rot input; k1 output; sis input; k2 output
function [k1, k2] = func_gen_K(symbol_q_rot, symbol_i_rot, sis)
% -------------------------------------------------------------------------
% Function gen_K
% -------------------------------------------------------------------------
    real_tmp = abs(symbol_i_rot);
    imag_tmp = abs(symbol_q_rot);
    
    % Determina quien es mayor la parte real o imaginaria
    if (real_tmp < imag_tmp)
        tmp = 1;
    else
        tmp = 0;
    end

    nt = numerictype(1,16,14);
    fm = hdlfimath;
    
    % calcula k1 y k2 
    if (sis == 1)
       k2 = fi(0, nt, fm);
    elseif (sis == 3 && tmp == 0)
       k2 = fi(sqrt(2)-1, nt, fm);
    else
       k2 = fi(1, nt, fm);
    end

    if (sis == 3 && tmp == 1)
       k1 = fi(sqrt(2)-1, nt, fm);
    else
       k1 = fi(1, nt, fm);
    end
end
% -------------------------------------------------------------------------

== matlab function cc_simulink/CC_FX/rotation/func_rot ==
  data: run input; sis input; val_in input; rot_real output; init_par input; rot_imag output
function [rot_real, rot_imag] = func_rot(run, sis, val_in, init_par)
% -------------------------------------------------------------------------
% Function rot
% -------------------------------------------------------------------------
    %#codegen
    persistent parity;
    if isempty(parity)
        parity = false; 
    end

    if (run == 0)
       parity = false;
    elseif (init_par == 1)
        parity = true;
    elseif (val_in == 1)
       parity = not(parity);
    end

    if (sis==1 && parity) % par
       rot_real = 0;  
       rot_imag = 1;
    elseif (sis==2 && not(parity)) % par
       rot_real = cos(pi/4);  
       rot_imag = sin(pi/4);
    elseif (sis==3 && not(parity)) % par
       rot_real = cos(pi/8);  
       rot_imag = sin(pi/8);
    else
       rot_real = 1;  
       rot_imag = 0;
    end 
end
% -------------------------------------------------------------------------

== matlab function cc_simulink/CC_FP/Subsystem/func_rd ==
  data: empty input; run input; val_err input; rd output; last_out output; rdy_in input
function [rd, last_out] = func_rd(empty, run, val_err, rdy_in)
% -------------------------------------------------------------------------
% Function valid
% -------------------------------------------------------------------------
    % persistent variable for the state 
    persistent ptr;
    if isempty(count)
        count = uint16(0);
    end

    % persistent variable for the state 
    persistent count_dwell;
    if isempty(count_dwell)
        count_dwell = uint8(0);
    end

    persistent add_pilot;
    if isempty(add_pilot)
        add_pilot = false;
    end

    % dwell symbol counter
    if (not(run) || (val_in && (last_in || count > uint16(946))))
         count = uint16(0);
    elseif (val_in)
        count = count + uint16(1);
    end

    % dwell number counter 
    if (not(run) || (val_in && (last_in || count > uint16(946))))
        count_dwell = uint8(0);
    elseif (val_in && count == uint16(946))
        count_dwell = count_dwell + uint8(1);
    end

    % generate the add pilot
    if (not(run) || (val_in && (last_in || count > uint16(946))))
       add_pilot = false; 
    elseif (count == uint16(64+32) || ...
            count == uint16(64+32+11) || ...
            count == uint16(64+32+11+157) || ...
            count == uint16(64+32+11+157+11) || ...
            count == uint16(64+32+11+157+11+157) || ...
            count == uint16(64+32+11+157+11+157+11) || ...
            count == uint16(64+32+11+157+11+157+11+157) || ...
            count == uint16(64+32+11+157+11+157+11+157+11) || ...
            count == uint16(64+32+11+157+11+157+11+157+11+157) || ...
            count == uint16(64+32+11+157+11+157+11+157+11+157+11) || ...
            count == uint16(64+32+11+157+11+157+11+157+11+157+11+157) || ...
            count == uint16(64+32+11+157+11+157+11+157+11+157+11+157+11))

        add_pilot = not(add_pilot);
    end
    

    % calculate last
    if (count_dwell == uint8(4) && count == uint16(935))
        last_out = true;
    else
        last_out = false;
    end

    % calculate last
    if (count == uint16(946) && val_in)
        init_par_int = true;
    else
        init_par_int = false;
    end

    val_out = mask_int && val_in;
    init_par = init_par_int && val_in;

end 
% -------------------------------------------------------------------------
